simulink model "MotorModel"  (R2021a)
settings: Solver=VariableStepAuto  StartTime=0.0  StopTime=0.4  RelTol=1e-3
model workspace (MAT data in the model file):
  J = 0.003408
  Ke = 0.0796
  Kt = 0.079
  La = 4.55e-05
  Ra = 0.06
  Tm = 1
  kf = 0.0001
settings Model: Creator=js20164  LastModifiedBy=james
settings SolverCC: AlgebraicLoopSolver=TrustRegion
settings DebuggingCC: SFMachineParentedDataDiag=warning

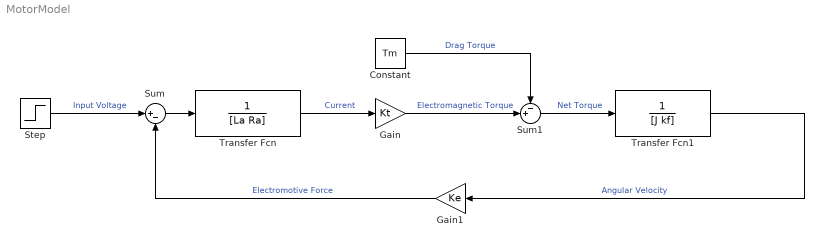
== system MotorModel ==
  Constant : Constant  Value=Tm
  Gain : Gain  Gain=Kt
  Gain1 : Gain  Gain=Ke
  Step : Step  Time=0.1  SampleTime=0
  Sum : Sum  Inputs=|+-
  Sum1 : Sum  Inputs=-+|
  Transfer Fcn : TransferFcn  Denominator=[La Ra]
  Transfer Fcn1 : TransferFcn  Denominator=[J kf]
  wires:
  Step/1 -> Sum/1  "Input Voltage"
  Sum/1 -> Transfer Fcn/1
  Transfer Fcn/1 -> Gain/1  "Current"
  Gain/1 -> Sum1/2  "Electromagnetic Torque"
  Sum1/1 -> Transfer Fcn1/1  "Net Torque"
  Transfer Fcn1/1 -> Gain1/1  "Angular Velocity"
  Gain1/1 -> Sum/2  "Electromotive Force"
  Constant/1 -> Sum1/1  "Drag Torque"
